simulink model "ExtendedErrorSpaceSim"  (R2020b)
settings: Solver=VariableStepAuto  StartTime=0.0  StopTime=3  RelTol=1e-3
undefined symbols (not defined in the file or in its folder): daq, drv, ees, gbox, mech, mld, mot, rads2rpm, sens
settings Model: Creator=Utente  LastModifiedBy=Utente

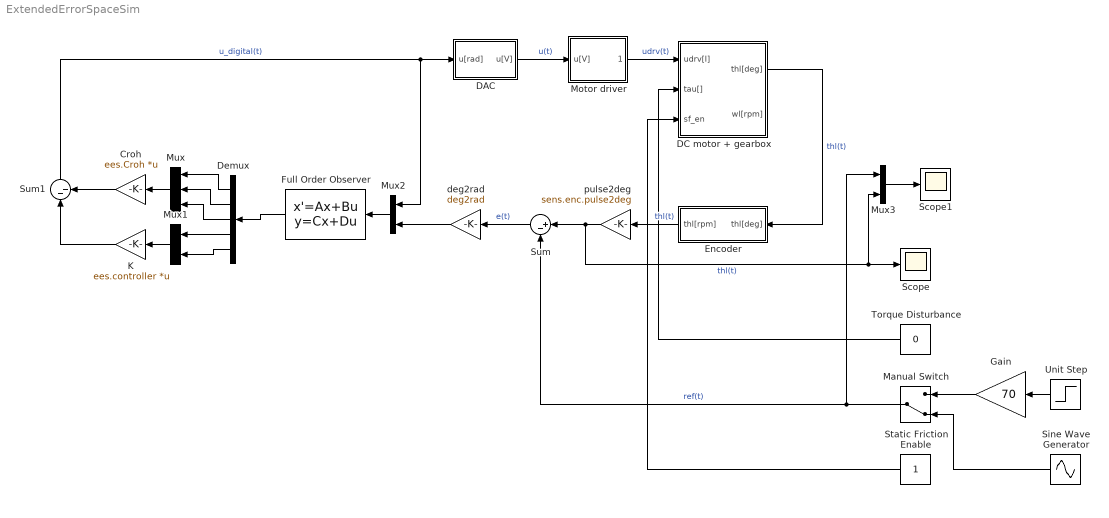
== system ExtendedErrorSpaceSim ==
  Croh : Gain  Gain=ees.Croh  Multiplication=Matrix(K*u)
  DAC : Subsystem
  DC motor + gearbox : Subsystem
  Demux : Demux  Outputs=5
  Encoder : Subsystem
  Full Order Observer : StateSpace  A=ees.Ae3 - ees.estimator3.Le*ees.Ce  B=[ees.Be, ees.estimator3.Le]  C=eye(5)  D=[0,0;0,0;0,0;0,0;0,0]  InitialCondition=0
  Gain : Gain  Gain=70
  K : Gain  Gain=ees.controller  Multiplication=Matrix(K*u)
  Manual Switch : ManualSwitch  CurrentSetting=0
  Motor driver : Subsystem
  Mux : Mux  Inputs=3
  Mux1 : Mux  Inputs=2
  Mux2 : Mux  Inputs=2
  Mux3 : Mux  Inputs=2
  Scope : Scope
  Scope1 : Scope
  Sine Wave Generator : Sin  Amplitude=40  Frequency=ees.controller3.w0
  Static Friction Enable : Constant
  Sum : Sum  Inputs=|+-
  Sum1 : Sum  Inputs=|--
  Torque Disturbance : Constant  Value=0
  Unit Step : Step  Time=0  SampleTime=0
  deg2rad : Gain  Gain=deg2rad
  pulse2deg : Gain  Gain=sens.enc.pulse2deg
  wires:
  Demux/3 -> Mux/3
  Demux/4 -> Mux1/1
  Demux/5 -> Mux1/2
  Demux/2 -> Mux/2
  Demux/1 -> Mux/1
  Full Order Observer/1 -> Demux/1
  Mux/1 -> Croh/1
  Sum1/1 -> Mux2/1, DAC/1(u[rad])  "u_digital(t)"
  Encoder/1(thl[rpm]) -> pulse2deg/1  "thl(t)"
  Motor driver/1(udrv[I]) -> DC motor + gearbox/1(udrv[I])  "udrv(t)"
  DAC/1(u[V]) -> Motor driver/1(u[V])  "u(t)"
  pulse2deg/1 -> Mux3/2, Scope/1, Sum/1  "thl(t)"
  DC motor + gearbox/1(thl[deg]) -> Encoder/1(thl[deg])  "thl(t)"
  Mux2/1 -> Full Order Observer/1
  Manual Switch/1 -> Mux3/1, Sum/2  "ref(t)"
  Sum/1 -> deg2rad/1  "e(t)"
  Mux1/1 -> K/1
  K/1 -> Sum1/1
  Croh/1 -> Sum1/2
  Static Friction Enable/1 -> DC motor + gearbox/3(sf_en)
  Torque Disturbance/1 -> DC motor + gearbox/2(tau[])
  deg2rad/1 -> Mux2/2
  Mux3/1 -> Scope1/1
  Unit Step/1 -> Gain/1
  Gain/1 -> Manual Switch/1
  Sine Wave Generator/1 -> Manual Switch/2

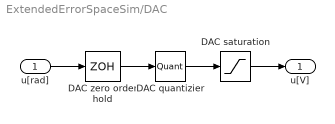
== system ExtendedErrorSpaceSim/DAC ==
  u[rad] : Inport
  DAC quantizier : Quantizer  QuantizationInterval=daq.dac.q
  DAC saturation : Saturate  UpperLimit=daq.dac.vdd  LowerLimit=daq.dac.vss
  DAC zero order hold : ZeroOrderHold  SampleTime=daq.dac.T_s
  u[V] : Outport
  wires:
  DAC quantizier/1 -> DAC saturation/1
  DAC zero order hold/1 -> DAC quantizier/1
  DAC saturation/1 -> u[V]/1
  u[rad]/1 -> DAC zero order hold/1

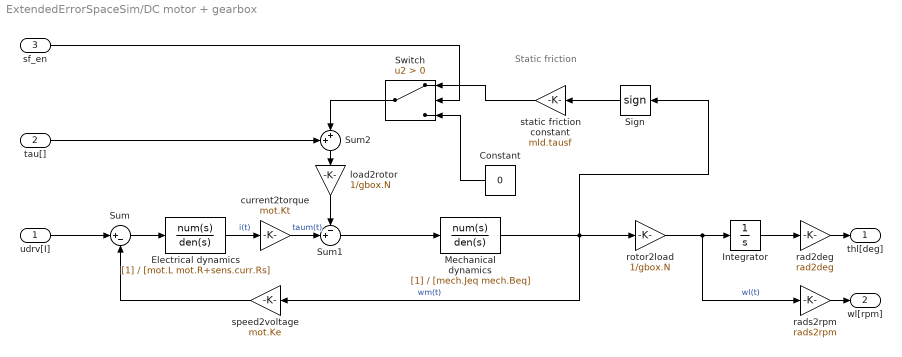
== system ExtendedErrorSpaceSim/DC motor + gearbox ==
  note: Static friction
  udrv[I] : Inport  Unit=V
  tau[] : Inport  Port=2  Unit=V
  sf_en : Inport  Port=3  Unit=V
  Constant : Constant  Value=0
  Electrical dynamics : TransferFcn  Denominator=[mot.L mot.R+sens.curr.Rs]
  Integrator : Integrator
  Mechanical dynamics : TransferFcn  Denominator=[mech.Jeq mech.Beq]
  Sign : Signum  ZeroCross=off
  Sum : Sum  Inputs=|+-
  Sum1 : Sum  Inputs=-+|
  Sum2 : Sum  Inputs=++|
  Switch : Switch  Criteria=u2 > Threshold
  current2torque : Gain  Gain=mot.Kt
  load2rotor : Gain  Gain=1/gbox.N
  rad2deg : Gain  Gain=rad2deg
  rads2rpm : Gain  Gain=rads2rpm
  rotor2load : Gain  Gain=1/gbox.N
  speed2voltage : Gain  Gain=mot.Ke
  static friction constant : Gain  Gain=mld.tausf
  thl[deg] : Outport  Unit=deg
  wl[rpm] : Outport  Port=2  Unit=rpm
  wires:
  load2rotor/1 -> Sum1/1
  Mechanical dynamics/1 -> Sign/1, rotor2load/1, speed2voltage/1  "wm(t)"
  Sign/1 -> static friction constant/1
  current2torque/1 -> Sum1/2  "taum(t)"
  Sum1/1 -> Mechanical dynamics/1
  speed2voltage/1 -> Sum/2
  rotor2load/1 -> rads2rpm/1, Integrator/1  "wl(t)"
  Electrical dynamics/1 -> current2torque/1  "i(t)"
  Integrator/1 -> rad2deg/1
  Sum/1 -> Electrical dynamics/1
  rads2rpm/1 -> wl[rpm]/1
  rad2deg/1 -> thl[deg]/1
  udrv[I]/1 -> Sum/1
  Sum2/1 -> load2rotor/1
  tau[]/1 -> Sum2/1
  Switch/1 -> Sum2/2
  static friction constant/1 -> Switch/1
  Constant/1 -> Switch/3
  sf_en/1 -> Switch/2

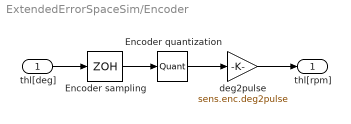
== system ExtendedErrorSpaceSim/Encoder ==
  thl[deg] : Inport
  Encoder quantization : Quantizer  QuantizationInterval=sens.enc.q
  Encoder sampling : ZeroOrderHold  SampleTime=sens.enc.T_s
  deg2pulse : Gain  Gain=sens.enc.deg2pulse
  thl[rpm] : Outport
  wires:
  Encoder quantization/1 -> deg2pulse/1
  deg2pulse/1 -> thl[rpm]/1
  Encoder sampling/1 -> Encoder quantization/1
  thl[deg]/1 -> Encoder sampling/1

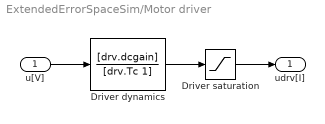
== system ExtendedErrorSpaceSim/Motor driver ==
  u[V] : Inport
  Driver dynamics : TransferFcn  Numerator=[drv.dcgain]  Denominator=[drv.Tc 1]
  Driver saturation : Saturate  UpperLimit=drv.vp  LowerLimit=drv.vm
  udrv[I] : Outport
  wires:
  Driver saturation/1 -> udrv[I]/1
  Driver dynamics/1 -> Driver saturation/1
  u[V]/1 -> Driver dynamics/1
